simulink model "Simulink_model"  (R2022b)
settings: Solver=VariableStepAuto  StartTime=0.0  StopTime=50  RelTol=1e-3
values from neighbouring files (symbols this model uses):
  D = 0.210    (= 0.21)    [input_data.m]
  DOWN_TH = readmatrix('DOWN_TH.xlsx')    [input_data.m]
  ENGINE_MAP = readmatrix('ENGINE_MAP.xlsx')    [input_data.m]
  Iei = 0.3    [input_data.m]
  Iv = 160    [input_data.m]
  Mt = 7000    [input_data.m]
  r_w = Rw*0.3    (= 0.36)    [input_data.m]
  Rfd = 4.4    [input_data.m]
  rload0 = f*G    (= 454.203)    [input_data.m]
  rload2 = Cx*ro*S    (= 1.5216)    [input_data.m]
  Ro_Lmbd = readmatrix('Ro_Lmbd.xlsx')    [input_data.m]
  Rw = 1.2    [input_data.m]
  SpeedRatio = readmatrix('SpeedRatio.xlsx')    [input_data.m]
  TABLE_DOWN = readmatrix('TABLE_DOWN.xlsx')    [input_data.m]
  TABLE_UP = readmatrix('TABLE_UP.xlsx')    [input_data.m]
  TH_VECTOR = readmatrix('TH_VECTOR.xlsx')    [input_data.m]
  TorqueRatio = readmatrix('TorqueRatio.xlsx')    [input_data.m]
  UP_TH = readmatrix('UP_TH.xlsx')    [input_data.m]
  V0 = 0.0    (= 0)    [input_data.m]
  WE_VECTOR = readmatrix('WE_VECTOR.xlsx')    [input_data.m]
undefined symbols (not defined in the file or in its folder): sigbuilder_block
settings Model: Creator=student-GM301  LastModifiedBy=EGOWKINGS
settings SolverCC: MaxConsecutiveMinStep=10  AlgebraicLoopSolver=TrustRegion
settings DebuggingCC: UnconnectedInputMsg=warning  UnconnectedOutputMsg=warning  UnconnectedLineMsg=warning  SFMachineParentedDataDiag=warning
settings ModelReferenceCC: EnableRefExpFcnMdlSchedulingChecks=on
settings RTWCC: DLArmComputeVersion=19.05

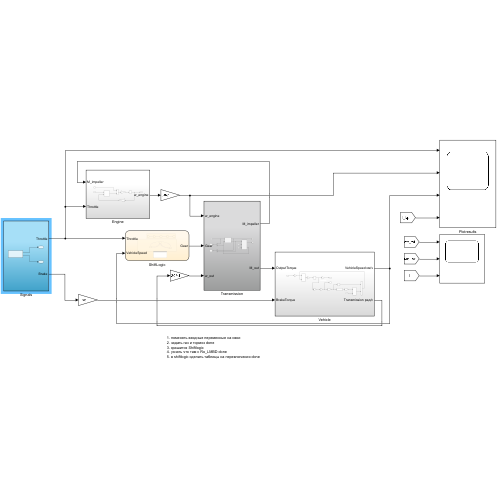
[thumbnail: Simulink's stored preview of the top-level diagram]
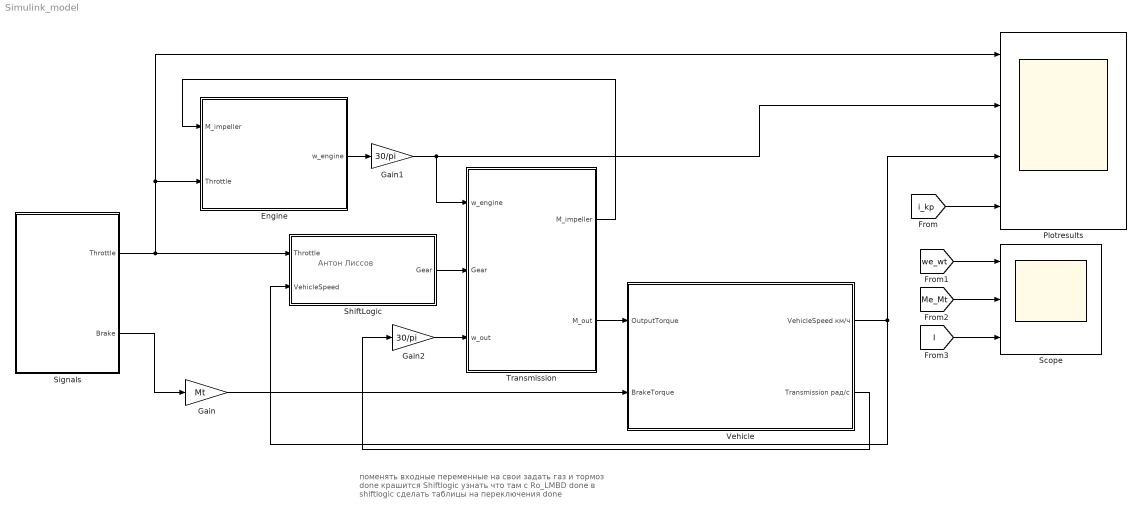
== system Simulink_model ==
  note: Антон Лисcов
  note: поменять входные переменные на свои
      | задать газ и тормоз done
      | крашится Shiftlogic
      | узнать что там с Ro_LMBD done
      | в shiftlogic сделать таблицы на переключения done
  Engine : Subsystem
  Gain : Gain  Gain=Mt
  Gain1 : Gain  Gain=30/pi
  Gain2 : Gain  Gain=30/pi
  Plotresults : Scope  NumInputPorts=4
  Scope : Scope  NumInputPorts=3
  ShiftLogic : Stateflow chart  TreatAsAtomicUnit=on
  Signals : Subsystem
  Transmission : Subsystem
  Vehicle : Subsystem
  wires:
  Signals/1(Throttle) -> Plotresults/1, Engine/2(Throttle), ShiftLogic/1(Throttle)
  Signals/2(Brake) -> Gain/1
  Gain/1 -> Vehicle/2(BrakeTorque)
  Transmission/2(M_out) -> Vehicle/1(OutputTorque)
  Engine/1(w_engine) -> Gain1/1
  Gain1/1 -> Transmission/1(w_engine), Plotresults/2
  Transmission/1(M_impeller) -> Engine/1(M_impeller)
  ShiftLogic/1(Gear) -> Transmission/2(Gear)
  Gain2/1 -> Transmission/3(w_out)
  Vehicle/2(Transmission рад/с) -> Gain2/1
  Vehicle/1(VehicleSpeed км/ч) -> ShiftLogic/2(VehicleSpeed), Plotresults/3
  [i_kp] -> Plotresults/4
  [I] -> Scope/3
  [Me_Mt] -> Scope/2
  [we_wt] -> Scope/1

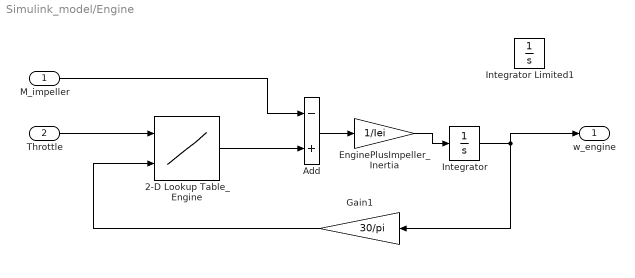
== system Simulink_model/Engine ==
  M_impeller : Inport
  Throttle : Inport  Port=2
  2-D Lookup Table_Engine : Lookup_n-D  BreakpointsForDimension1=TH_VECTOR  BreakpointsForDimension2=WE_VECTOR  Table=ENGINE_MAP  InternalRulePriority=Speed  RndMeth=Simplest
      settings: InputPortMap=u0,u1
  Add : Sum  Inputs=-+
  EnginePlusImpeller_Inertia : Gain  Gain=1/Iei
  Gain1 : Gain  Gain=30/pi
  Integrator : Integrator  InitialCondition=105  UpperSaturationLimit=6500  LowerSaturationLimit=500  ZeroCross=off
  Integrator Limited1 : Integrator  InitialCondition=1000  LimitOutput=on  UpperSaturationLimit=6000  LowerSaturationLimit=600  ZeroCross=off
  w_engine : Outport
  wires:
  Throttle/1 -> 2-D Lookup Table_Engine/1
  M_impeller/1 -> Add/1
  2-D Lookup Table_Engine/1 -> Add/2
  Add/1 -> EnginePlusImpeller_Inertia/1
  EnginePlusImpeller_Inertia/1 -> Integrator/1
  Integrator/1 -> w_engine/1, Gain1/1
  Gain1/1 -> 2-D Lookup Table_Engine/2

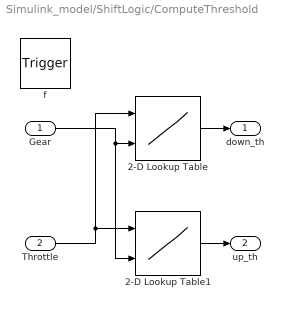
== system Simulink_model/ShiftLogic/ComputeThreshold ==
  Gear : Inport  OutDataTypeStr=double  PortDimensions=1
  Throttle : Inport  Port=2  OutDataTypeStr=double  PortDimensions=1
  f : TriggerPort  TriggerType=function-call  VariantControl=(inherit)
      settings: CopyFcn=Stateflow.SLINSF.SimulinkMan.removeBlockPreDeleteFcn  PreDeleteFcn=Stateflow.SLINSF.SimulinkMan.unsafePredeleteFcn
  2-D Lookup Table : Lookup_n-D  BreakpointsForDimension1=DOWN_TH  BreakpointsForDimension2=[1:5]  Table=TABLE_DOWN  InternalRulePriority=Speed  RndMeth=Simplest
      settings: InputPortMap=u0,u1
  2-D Lookup Table1 : Lookup_n-D  BreakpointsForDimension1=UP_TH  BreakpointsForDimension2=[1:5]  Table=TABLE_UP  InternalRulePriority=Speed  RndMeth=Simplest
      settings: InputPortMap=u0,u1
  down_th : Outport
  up_th : Outport  Port=2
  wires:
  2-D Lookup Table/1 -> down_th/1
  2-D Lookup Table1/1 -> up_th/1
  Throttle/1 -> 2-D Lookup Table/1, 2-D Lookup Table1/1
  Gear/1 -> 2-D Lookup Table1/2, 2-D Lookup Table/2

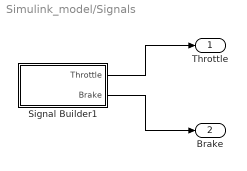
== system Simulink_model/Signals ==
  Signal Builder1 : Subsystem  Tag=STV Subsys  LoadFcn=sigbuilder_block('load');  StartFcn=sigbuilder_block('start');  StopFcn=sigbuilder_block('stop');  ClipboardFcn=sigbuilder_block('clipboard');  mask(Sigbuilder block){tuvar=[0:10]}
      mask help: Simulink:masks:SigbuilderBlock_MD
      mask init:
      | if ~strcmp(get_param(bdroot(gcbh),'SimulationStatus'),'stopped') tuvar = sigbuilder_block('maskInit'); end
      settings: CopyFcn=sigbuilder_block('copy');  DeleteFcn=sigbuilder_block('delete');  ModelCloseFcn=sigbuilder_block('modelClose');  PreSaveFcn=sigbuilder_block('preSave');  PauseFcn=sigbuilder_block('pause');  ContinueFcn=sigbuilder_block('continue');  NameChangeFcn=sigbuilder_block('namechange');  OpenFcn=sigbuilder_block('open',[97.2 83.4 550.8 400.2 ]);  CloseFcn=sigbuilder_block('close');
      mask Display: plot(0, 0, 100, 100,[2, 2, 32, 32, 2], [68, 8, 8, 68, 68],[32, 2], [38, 38], [32, 19, 2],[53, 60, 44], [32, 17, 17, 2],[16, 16, 31, 31]);txt = getActiveGroup(gcbh);text(2, 100, txt,'verticalAlignment', 'top');
  Throttle : Outport
  Brake : Outport  Port=2
  wires:
  Signal Builder1/1(Throttle) -> Throttle/1
  Signal Builder1/2(Brake) -> Brake/1

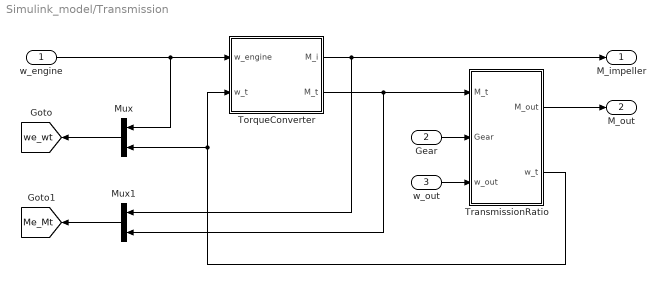
== system Simulink_model/Transmission ==
  w_engine : Inport
  Gear : Inport  Port=2
  w_out : Inport  Port=3
  Mux : Mux  Inputs=2
  Mux1 : Mux  Inputs=2
  TorqueConverter : Subsystem
  TransmissionRatio : Subsystem
  M_impeller : Outport
  M_out : Outport  Port=2
  tag scope: Me_Mt=global, we_wt=global
  wires:
  w_engine/1 -> Mux/1, TorqueConverter/1(w_engine)
  Mux/1 -> [we_wt]
  Mux1/1 -> [Me_Mt]
  TransmissionRatio/1(M_out) -> M_out/1
  TorqueConverter/1(M_i) -> Mux1/1, M_impeller/1
  Gear/1 -> TransmissionRatio/2(Gear)
  w_out/1 -> TransmissionRatio/3(w_out)
  TorqueConverter/2(M_t) -> Mux1/2, TransmissionRatio/1(M_t)
  TransmissionRatio/2(w_t) -> Mux/2, TorqueConverter/2(w_t)

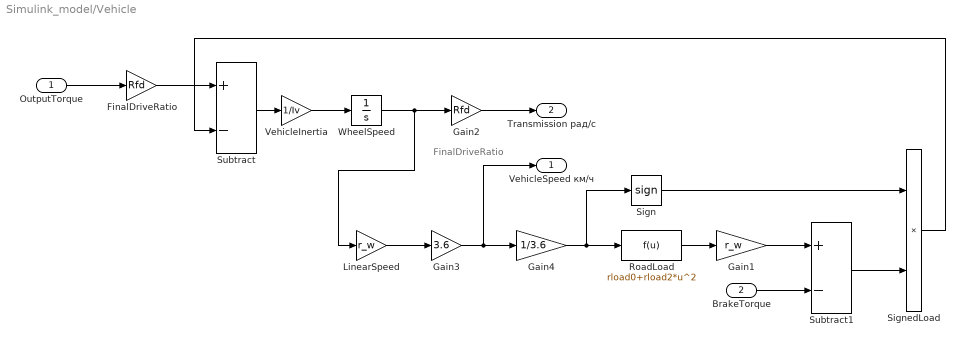
== system Simulink_model/Vehicle ==
  note: FinalDriveRatio
  OutputTorque : Inport
  BrakeTorque : Inport  Port=2
  FinalDriveRatio : Gain  Gain=Rfd
  Gain1 : Gain  Gain=r_w
  Gain2 : Gain  Gain=Rfd
  Gain3 : Gain  Gain=3.6
  Gain4 : Gain  Gain=1/3.6
  LinearSpeed : Gain  Gain=r_w
  RoadLoad : Fcn  Expr=rload0+rload2*u^2
  Sign : Signum
  SignedLoad : Product
  Subtract : Sum  Inputs=+-
  Subtract1 : Sum  Inputs=+-
  VehicleInertia : Gain  Gain=1/Iv
  WheelSpeed : Integrator  InitialCondition=V0/Rw  ZeroCross=off
  VehicleSpeed км/ч : Outport
  Transmission рад/с : Outport  Port=2
  wires:
  OutputTorque/1 -> FinalDriveRatio/1
  FinalDriveRatio/1 -> Subtract/1
  Subtract/1 -> VehicleInertia/1
  VehicleInertia/1 -> WheelSpeed/1
  WheelSpeed/1 -> LinearSpeed/1, Gain2/1
  Gain2/1 -> Transmission рад/с/1
  LinearSpeed/1 -> Gain3/1
  Gain3/1 -> VehicleSpeed км/ч/1, Gain4/1
  Gain4/1 -> RoadLoad/1, Sign/1
  RoadLoad/1 -> Gain1/1
  Gain1/1 -> Subtract1/1
  BrakeTorque/1 -> Subtract1/2
  Sign/1 -> SignedLoad/1
  Subtract1/1 -> SignedLoad/2
  SignedLoad/1 -> Subtract/2

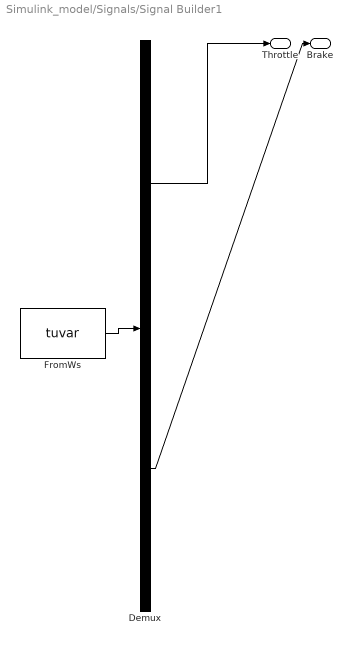
== system Simulink_model/Signals/Signal Builder1 ==
  Demux : Demux  Tag=STV Demux  Outputs=2
      settings: DisplayOption=none
  FromWs : FromWorkspace  Tag=STV FromWs  VariableName=tuvar
      SigBuilderData=|
      | common.afterFinalStr = 'Extrapolate'
      | common.sampleTime = 0
      | dataSet.timeRange = [0 50]
      | dataSet.name = 'Group 1'
      | sbobj.Groups.Name = 'Group 1'
      | sbobj.Groups.Signals(1).Name = 'Throttle'
      | sbobj.Groups.Signals(1).XData = [0 15 15 50]
      | sbobj.Groups.Signals(1).YData = [60 30 100 67]
      | sbobj.Groups.Signals(2).Name = 'Brake'
      | sbobj.Groups.Signals(2).XData = [0 50]
      | sbobj.Groups.Signals(2).YData = [0 0]
      | sbobj.Groups.TimeRange = [0 50]
  Throttle : Outport  Tag=STV Outport
  Brake : Outport  Tag=STV Outport  Port=2
  wires:
  Demux/1 -> Throttle/1
  FromWs/1 -> Demux/1
  Demux/2 -> Brake/1

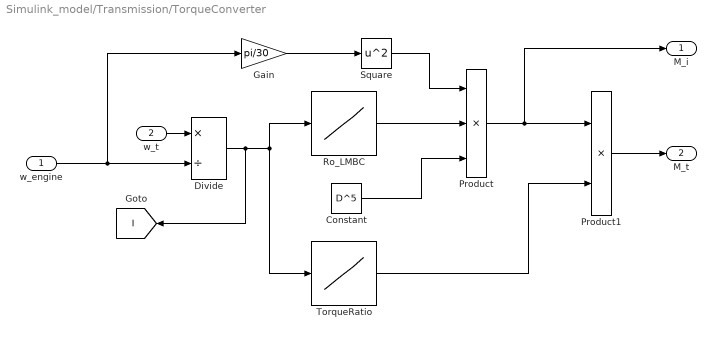
== system Simulink_model/Transmission/TorqueConverter ==
  w_engine : Inport
  w_t : Inport  Port=2
  Constant : Constant  Value=D^5
  Divide : Product  Inputs=*/
  Gain : Gain  Gain=pi/30
  Product : Product  Inputs=3
  Product1 : Product
  Ro_LMBC : Lookup_n-D  NumberOfTableDimensions=1  BreakpointsForDimension1=SpeedRatio  Table=Ro_Lmbd  InternalRulePriority=Speed  RndMeth=Simplest
  Square : Math  Operator=square
  TorqueRatio : Lookup_n-D  NumberOfTableDimensions=1  BreakpointsForDimension1=SpeedRatio  Table=TorqueRatio  InternalRulePriority=Speed  RndMeth=Simplest
  M_i : Outport
  M_t : Outport  Port=2
  tag scope: I=global
  wires:
  Gain/1 -> Square/1
  w_t/1 -> Divide/1
  w_engine/1 -> Divide/2, Gain/1
  Square/1 -> Product/1
  Ro_LMBC/1 -> Product/2
  Divide/1 -> [I], TorqueRatio/1, Ro_LMBC/1
  TorqueRatio/1 -> Product1/2
  Product/1 -> M_i/1, Product1/1
  Product1/1 -> M_t/1
  Constant/1 -> Product/3

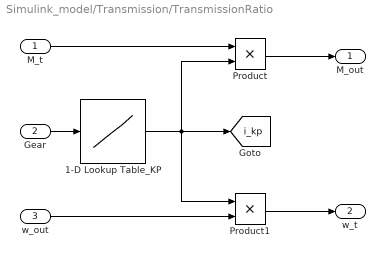
== system Simulink_model/Transmission/TransmissionRatio ==
  M_t : Inport
  Gear : Inport  Port=2
  w_out : Inport  Port=3
  1-D Lookup Table_KP : Lookup_n-D  NumberOfTableDimensions=1  BreakpointsForDimension1=[1 2 3 4 5]  Table=[4.65 2.596 1.526 1.000 0.856]  InterpMethod=Nearest  ExtrapMethod=Clip  InternalRulePriority=Speed  RndMeth=Simplest
  Product : Product
  Product1 : Product
  M_out : Outport
  w_t : Outport  Port=2
  tag scope: i_kp=global
  wires:
  w_out/1 -> Product1/2
  M_t/1 -> Product/1
  Product/1 -> M_out/1
  Product1/1 -> w_t/1
  Gear/1 -> 1-D Lookup Table_KP/1
  1-D Lookup Table_KP/1 -> Product1/1, Product/2, [i_kp]

== stateflow chart Simulink_model/ShiftLogic ==
  settings: updateMethod=DISCRETE  sampleTime=0.04
  state gear_state/ [parallel]
    settings: executionOrder=1
    state first
      entry:
      Gear = 1;
    state second
      entry:
      Gear = 2;
    state third
      entry:
      Gear = 3;
    state fourth
      entry:
      Gear = 4;
    state fifth
      entry:
      Gear = 5;
    (default) -> first
    second -> third [order 1] : UP
    third -> fourth [order 1] : UP
    fourth -> fifth [order 1] : UP
    first -> second : UP
    second -> first [order 2] : DOWN
    third -> second [order 2] : DOWN
    fourth -> third [order 2] : DOWN
    fifth -> fourth : DOWN
  state selection_state [parallel]
    during:
    [down_th, up_th] = ComputeThreshold(Gear, Throttle);
    settings: executionOrder=2
    state steady_state
    state downshifting
    state upshifting
    (default) -> steady_state
    steady_state -> downshifting [order 2] : [VehicleSpeed < down_th]
    steady_state -> upshifting [order 1] : [VehicleSpeed > up_th]
    downshifting -> steady_state [order 2] : [VehicleSpeed > down_th]
    downshifting -> steady_state [order 1] : after(TWAIT, tick)
        | [VehicleSpeed <= down_th]
        | {gear_state.DOWN}
    upshifting -> steady_state [order 1] : after(TWAIT, tick)
        | [VehicleSpeed >= up_th]
        | {gear_state.UP}
    upshifting -> steady_state [order 2] : [VehicleSpeed < up_th]
  state [down_th, up_th] = ComputeThreshold(Gear, Throttle) [function]
  data: Gear function_input double size=1; Throttle function_input double size=1; down_th function_output; up_th function_output; Throttle input double; VehicleSpeed input double; Gear output fixdt(0,8,5) [1..5]; TWAIT parameter fixdt(0,8,6); down_th local double; up_th local double
  events: UP local RISING_EDGE_EVENT; DOWN local RISING_EDGE_EVENT
